simulink model "wgn_generator"  (R2019a)
settings: Solver=VariableStepAuto  StartTime=0.0  StopTime=10.0  RelTol=1e-10
libraries: simulink x1
settings Model: Creator=USER  LastModifiedBy=USER

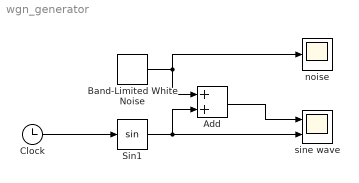
== system wgn_generator ==
  Add : Sum
  Band-Limited White Noise : simulink/Sources/Band-Limited White Noise  Cov=[1E-7]  Ts=0.001  seed=[23341]
  Clock : Clock
  Sin1 : Trigonometry
  noise : Scope
  sine wave : Scope  NumInputPorts=2
  wires:
  Clock/1 -> Sin1/1
  Band-Limited White Noise/1 -> noise/1, Add/1
  Sin1/1 -> sine wave/2, Add/2
  Add/1 -> sine wave/1
